simulink model "BPSK"  (R2015a)
settings: Solver=ode45  StartTime=0.0  StopTime=1e3  RelTol=1e-3
libraries: commdigbbndpm3 x2, commchan3 x1, commsink2 x1, commrandsrc2 x1
settings Model: Creator=levyg  LastModifiedBy=levyg

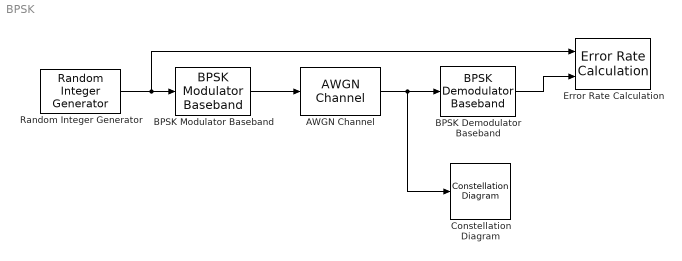
== system BPSK ==
  AWGN Channel : commchan3/AWGN Channel  InputProcessing=Columns as channels (frame based)  seed=67  noiseMode="Signal to noise ratio  (Eb/No)"  EbNodB=EbN0  EsNodB=10  SNRdB=10  bitsPerSym=1  Ps=1  Tsym=0.5  variance=1
  BPSK Demodulator Baseband : commdigbbndpm3/BPSK Demodulator Baseband  Ph=0  DecType=Hard decision  VarSource=Dialog  Variance=1  outDtype=Inherit via internal rule  derotateFactorWordLen=16
  BPSK Modulator Baseband : commdigbbndpm3/BPSK Modulator Baseband  Ph=0  outDtype=double  outWordLen=16  outUDDataType=sfix(16)  outFracLenMode=Best precision  outFracLen=15
  Constellation Diagram : ConstellationDiagram
  Error Rate Calculation : commsink2/Error Rate Calculation  N=0  st_delay=0  cp_mode=Entire frame  subframe=[]  PMode=Workspace  WsName=ErrorVec  RsMode2=off  stop=off  numErr=100  maxBits=1e6
  Random Integer Generator : commrandsrc2/Random Integer Generator  mul=2  seed=37  Ts=0.5  frameBased=on  sampPerFrame=1e6  orient=off  outDataType=double
  wires:
  BPSK Modulator Baseband/1 -> AWGN Channel/1
  AWGN Channel/1 -> Constellation Diagram/1, BPSK Demodulator Baseband/1
  Random Integer Generator/1 -> Error Rate Calculation/1, BPSK Modulator Baseband/1
  BPSK Demodulator Baseband/1 -> Error Rate Calculation/2
